simulink library "CryoDetLibCMB"  (R2016b)
settings: Solver=VariableStepAuto  StartTime=0.0  StopTime=10.0  RelTol=1e-3
undefined symbols (not defined in the file): A, B, C, D, Fadc, Fclk, PCIN, xlipgetpartsetting
libraries: xbsIndex_r4 x640, CryoDetLibCMB x81, CryoDetLib x2, simulink x1
(part 7 of 12)

== system CryoDetLibCMB/Loop Filter1 ==
  note: loop filter takes frequency word in, creates frequency word out with setpoint frequency, amplitude
  note: loopFilter
      | multi-line feedback block
      | mplement intial frequency, limits, integrator, gain
  note: F out should be Fi + DF
      | where DF is integral of frequency error dF subject to limits and FBen
  note: Saturate dF at +-FBlimit
  valid : Inport
  feedbackPolarity : Inport  Port=2
  feedbackGain : Inport  Port=3
  feedbackLimitHi : Inport  Port=4
  feedbackLimitLo : Inport  Port=5
  freqError : Inport  Port=6
  freqWord : Inport  Port=7
  ch : Inport  Port=8
  reset : Inport  Port=9
  AddSub1 : xbsIndex_r4/AddSub  mode=Addition  use_carryin=off  use_carryout=off  en=off  latency=3  precision=User Defined  arith_type=Unsigned  n_bits=24  bin_pt=24  quantization=Truncate  overflow=Wrap  use_behavioral_HDL=off  hw_selection=Fabric  pipelined=on  dbl_ovrd=off  block_type=addsub
  BitBasher : xbsIndex_r4/BitBasher  bitexpr=out={fbEn, 3'b0, amp, freq}  display_expr=off  sr_1=out  arith_type1=Unsigned  bin_pt1=0  sr_2=2  arith_type2=Unsigned  bin_pt2=0  sr_3=3  arith_type3=Unsigned  bin_pt3=0  sr_4=4  arith_type4=Unsigned  bin_pt4=0  dbl_ovrd=off  block_type=bitbasher
  Concat1 : xbsIndex_r4/Concat  num_inputs=2  dbl_ovrd=off  block_type=concat
  Constant3 : xbsIndex_r4/Constant  const=0  gui_display_data_type=Fixed-point  arith_type=Signed (2's comp)  n_bits=32  bin_pt=30  preci_type=Single  exp_width=8  frac_width=24  explicit_period=off  period=1  equ=P=C  opselect=C  inp2=PCIN>>17  opr=+  inp1=P  carry=CIN  dbl_ovrd=off  block_type=constant
  Convert : xbsIndex_r4/Convert  gui_display_data_type=Fixed-point  arith_type="Signed  (2's comp)"  n_bits=32  bin_pt=30  float_type=Single  exp_bits=8  fraction_bits=24  quantization=Truncate  overflow=Wrap  en=off  latency=0  pipeline=off  dbl_ovrd=off  block_type=convert
  Convert1 : xbsIndex_r4/Convert  gui_display_data_type=Fixed-point  arith_type="Signed  (2's comp)"  n_bits=16  bin_pt=14  float_type=Single  exp_bits=8  fraction_bits=24  quantization=Truncate  overflow=Wrap  en=off  latency=0  pipeline=off  dbl_ovrd=off  block_type=convert
  Convert2 : xbsIndex_r4/Convert  gui_display_data_type=Fixed-point  arith_type="Signed  (2's comp)"  n_bits=48  bin_pt=37  float_type=Single  exp_bits=8  fraction_bits=24  quantization=Truncate  overflow=Wrap  en=off  latency=0  pipeline=off  dbl_ovrd=off  block_type=convert
  Convert3 : xbsIndex_r4/Convert  gui_display_data_type=Fixed-point  arith_type="Signed  (2's comp)"  n_bits=16  bin_pt=15  float_type=Single  exp_bits=8  fraction_bits=24  quantization=Truncate  overflow=Wrap  en=off  latency=0  pipeline=off  dbl_ovrd=off  block_type=convert
  Convert4 : xbsIndex_r4/Convert  gui_display_data_type=Fixed-point  arith_type="Signed  (2's comp)"  n_bits=16  bin_pt=15  float_type=Single  exp_bits=8  fraction_bits=24  quantization=Truncate  overflow=Wrap  en=off  latency=0  pipeline=off  dbl_ovrd=off  block_type=convert
  Convert5 : xbsIndex_r4/Convert  gui_display_data_type=Fixed-point  arith_type="Signed  (2's comp)"  n_bits=24  bin_pt=23  float_type=Single  exp_bits=8  fraction_bits=24  quantization=Truncate  overflow=Wrap  en=off  latency=0  pipeline=off  dbl_ovrd=off  block_type=convert
  "DSP48 Macro 3.0 " : xbsIndex_r4/DSP48 Macro 3.0   dsptype=Target XtremeDSP Slice: DSP48E2  instruction_list=A*B+C  AvailableInstructions=|  show_filtered=on  pipeline_options=Expert  dspimage=?  tier_1=off  tier_2=off  tier_3=off  tier_4=off  tier_5=off  tier_6=off  dreg_1=off  dreg_2=off  dreg_3=off  areg_1=off  areg_2=off  areg_3=on  areg_4=on  breg_1=off  breg_2=off  breg_3=on  breg_4=on  mreg_5=on  concatreg_3=off  concatreg_4=off  concatreg_5=off  creg_1=off  creg_2=off  creg_3=on  creg_4=on  creg_5=on  preg_6=on  cinreg_1=off  cinreg_2=off  cinreg_3=off  cinreg_4=off  cinreg_5=off  opreg_1=off  opreg_2=off  opreg_3=off  opreg_4=off  opreg_5=off  output_properties=Full_Precision  p_width=33  p_binarywidth=30  has_acout=off  has_bcout=off  has_pcout=off  has_carryout=off  has_carrycascout=off  has_ce=off  has_d_ce=off  has_a_ce=off  has_b_ce=off  has_concat_ce=off  has_c_ce=off  has_m_ce=off  has_p_ce=off  has_sel_ce=off  has_sclr=off  has_d_sclr=off  has_a_sclr=off  has_b_sclr=off  has_concat_sclr=off  has_c_sclr=off  has_m_sclr=off  has_p_sclr=off  has_sel_sclr=off  use_dsp48=on  simulation_type=fast_sim  simulation_model=sysgen:xbip_dsp48_macro_v3_0  gui_behaviour=Sysgen  instruction1='#'  ip_name=DSP48 Macro  ip_version=3.0  dsptool_ready=true  ipcore_usecache=true  ipcore_useipmodelcache=true  wrapper_available=true  port_translation_map={ 'ce' => 'en', 'sclr' => 'rst'}  ipcore_latency_function='has_combinational'  structural_sim=false  ipcore_verbose=false  ipcore_port_config={ 'carryin' => { 'arith' => 'ufix', 'binpt' => 0.00000000000, 'width' => 1.00000000000}, 'carrycascin' => { 'arith' => 'ufix', 'binpt' => 0.00000000000, 'width' => 1.00000000000}, 'carrycascout' => { 'arith' => 'ufix', 'binpt' => 0.00000000000, 'width' => 1.00000000000}, 'carryout' => { 'arith' => 'ufix', 'binpt' => 0.00000000000, 'width' => 1.00000000000}}  ipcore_xco_need_fpga_part=true  block_type=xbip_dsp48_macro_v3_0
      | -(A*B+C)
      | -(A*B+C+CARRYIN)
      | -(A*B+CARRYIN)
      | -(C+A*B+CARRYIN)
      | -(P+A*B+CARRYIN)
      | -C+A*B+C
      | -P+A*B+C
      | -P>>17+A*B+C
      | -PCIN+A*B+C
      | -PCIN>>17+A*B+C
      | A*B+C
      | A*B+C+C
      | A*B+C+C+CARRYIN
      | A*B+C+CARRYIN
      | A*B+C+P
      | A*B+C+P+CARRYIN
      | A*B+C+P>>17
      | A*B+C+P>>17+CARRYIN
      | A*B+C+PCIN
      | A*B+C+PCIN+CARRYIN
      | A*B+C+PCIN>>17
      | A*B+C+PCIN>>17+CARRYIN
      | A*B+C-C
      | A*B+C-P
      | A*B+C-P>>17
      | A*B+C-PCIN
      | A*B+C-PCIN>>17
      | A*B+CARRYIN
      | C+A*B+C
      | C+A*B+C+CARRYIN
      | C+A*B+CARRYIN
      | C+C+A*B+CARRYIN
      | C+P+A*B+CARRYIN
      | C+P>>17+A*B+CARRYIN
      | C+PCIN+A*B+CARRYIN
      | C+PCIN>>17+A*B+CARRYIN
      | C-(A*B+C)
      | C-(A*B+C+CARRYIN)
      | C-(A*B+CARRYIN)
      | C-(C+A*B+CARRYIN)
      | C-(P+A*B+CARRYIN)
      | P+A*B+C
      | P+A*B+C+CARRYIN
      | P+A*B+CARRYIN
      | P+C+A*B+CARRYIN
      | P+P+A*B+CARRYIN
      | P+P>>17+A*B+CARRYIN
      | P+PCIN+A*B+CARRYIN
      | P+PCIN>>17+A*B+CARRYIN
      | P-(A*B+C)
      | P-(A*B+C+CARRYIN)
      | P-(A*B+CARRYIN)
      | P-(C+A*B+CARRYIN)
      | P-(P+A*B+CARRYIN)
      | P>>17+A*B+C
      | P>>17+A*B+C+CARRYIN
      | P>>17+A*B+CARRYIN
      | P>>17+C+A*B+CARRYIN
      | P>>17+P+A*B+CARRYIN
      | P>>17-(A*B+C)
      | P>>17-(A*B+C+CARRYIN)
      | P>>17-(A*B+CARRYIN)
      | P>>17-(C+A*B+CARRYIN)
      | P>>17-(P+A*B+CARRYIN)
      | PCIN+A*B+C
      | PCIN+A*B+C+CARRYIN
      | PCIN+A*B+CARRYIN
      | PCIN+C+A*B+CARRYIN
      | PCIN+P+A*B+CARRYIN
      | PCIN-(A*B+C)
      | PCIN-(A*B+C+CARRYIN)
      | PCIN-(A*B+CARRYIN)
      | PCIN-(C+A*B+CARRYIN)
      | PCIN-(P+A*B+CARRYIN)
      | PCIN>>17+A*B+C
      | PCIN>>17+A*B+C+CARRYIN
      | PCIN>>17+A*B+CARRYIN
      | PCIN>>17+C+A*B+CARRYIN
      | PCIN>>17+P+A*B+CARRYIN
      | PCIN>>17-(A*B+C)
      | PCIN>>17-(A*B+C+CARRYIN)
      | PCIN>>17-(A*B+CARRYIN)
      | PCIN>>17-(C+A*B+CARRYIN)
      | PCIN>>17-(P+A*B+CARRYIN)
      | RNDMACC(A*B+C+P)
      | RNDSIMPLE(A*B+C)
      | RNDSIMPLE(A*B+C+CARRYIN)
      | RNDSIMPLE(A*B+CARRYIN)
      | RNDSIMPLE(C+A*B+CARRYIN)
      | RNDSIMPLE(P+A*B+CARRYIN)
      | RNDSIMPLE(P>>17+A*B+CARRYIN)
      | RNDSIMPLE(PCIN+A*B+CARRYIN)
      | RNDSIMPLE(PCIN>>17+A*B+CARRYIN)
      settings: infoedit=<html>Valid operands: CONCAT, P, C, PCIN, P>>17, PCIN>>17, CARRYIN, CARRYCASCIN, ACIN, A, BCIN,B<br><br>Valid operators: +, -, *, ()<br><br>Valid functions: RNDSIMPLE, RNDSYM<br><br>Instructions are case insensitive and tolerate spaces.</html>
  Delay : xbsIndex_r4/Delay  rst=off  infoeditControl=Selection of Reset will increase slice count due to use of real FFs and instead of SRLs  en=off  latency=121  reg_retiming=off  dbl_ovrd=off  block_type=delay
  Delay1 : xbsIndex_r4/Delay  rst=off  infoeditControl=Selection of Reset will increase slice count due to use of real FFs and instead of SRLs  en=off  latency=4  reg_retiming=off  dbl_ovrd=off  block_type=delay
  Delay2 : xbsIndex_r4/Delay  rst=off  infoeditControl=Selection of Reset will increase slice count due to use of real FFs and instead of SRLs  en=off  latency=3  reg_retiming=off  dbl_ovrd=off  block_type=delay
  Delay3 : xbsIndex_r4/Delay  rst=off  infoeditControl=Selection of Reset will increase slice count due to use of real FFs and instead of SRLs  en=off  latency=3  reg_retiming=off  dbl_ovrd=off  block_type=delay
  Delay4 : xbsIndex_r4/Delay  rst=off  infoeditControl=Selection of Reset will increase slice count due to use of real FFs and instead of SRLs  en=off  latency=3  reg_retiming=off  dbl_ovrd=off  block_type=delay
  Delay7 : xbsIndex_r4/Delay  rst=off  infoeditControl=Selection of Reset will increase slice count due to use of real FFs and instead of SRLs  en=off  latency=10  reg_retiming=off  dbl_ovrd=off  block_type=delay
  Delay8 : xbsIndex_r4/Delay  rst=off  infoeditControl=Selection of Reset will increase slice count due to use of real FFs and instead of SRLs  en=off  latency=10  reg_retiming=off  dbl_ovrd=off  block_type=delay
  Mux : xbsIndex_r4/Mux  inputs=2  en=off  latency=1  precision=User Defined  arith_type="Signed  (2's comp)"  n_bits=16  bin_pt=14  quantization=Truncate  overflow=Wrap  dbl_ovrd=off  block_type=mux
  Mux1 : xbsIndex_r4/Mux  inputs=2  en=off  latency=1  precision=Full  arith_type=Unsigned  n_bits=16  bin_pt=14  quantization=Truncate  overflow=Wrap  dbl_ovrd=off  block_type=mux
  Mux2 : xbsIndex_r4/Mux  inputs=3  en=off  latency=1  precision=Full  arith_type=Unsigned  n_bits=16  bin_pt=14  quantization=Truncate  overflow=Wrap  dbl_ovrd=off  block_type=mux
  Negate : xbsIndex_r4/Negate  precision=User Defined  arith_type="Signed  (2's comp)"  n_bits=16  bin_pt=15  quantization=Truncate  overflow=Wrap  en=off  latency=2  dbl_ovrd=off  block_type=negate
  Register3 : xbsIndex_r4/Register  init=0  rst=off  en=off  dbl_ovrd=off  block_type=register
  Relational3 : xbsIndex_r4/Relational  mode=a>b  op_type=Bool  en=off  latency=1  dbl_ovrd=off  block_type=relational
  Relational4 : xbsIndex_r4/Relational  mode=a<b  op_type=Bool  en=off  latency=1  dbl_ovrd=off  block_type=relational
  freqWordDecoder1 : CryoDetLibCMB/freqWordDecoder
  freqWordDecoder2 : CryoDetLibCMB/freqWordDecoder
  valid_o : Outport
  freqWordOut : Outport  Port=2
  ch_o : Outport  Port=3
  wires:
  Convert5/1 -> "DSP48 Macro 3.0 "/1
  freqError/1 -> Convert5/1
  Mux/1 -> "DSP48 Macro 3.0 "/2
  Convert4/1 -> Mux2/3, Relational4/1
  Convert3/1 -> Relational3/1, Mux2/4
  Convert1/1 -> Mux/2, Negate/1
  "DSP48 Macro 3.0 "/1 -> Convert/1
  Convert2/1 -> "DSP48 Macro 3.0 "/3
  Mux1/1 -> Relational3/2, Relational4/2, Register3/1
  Delay/1 -> Convert2/1
  Mux2/1 -> AddSub1/2, Delay/1
  Register3/1 -> Mux2/2
  feedbackLimitLo/1 -> Convert3/1
  Concat1/1 -> Mux2/1
  Relational4/1 -> Concat1/2
  Relational3/1 -> Concat1/1
  Constant3/1 -> Mux1/2
  Convert/1 -> Mux1/3
  freqWordDecoder1/1 -> Mux1/1
  Negate/1 -> Mux/3
  feedbackLimitHi/1 -> Convert4/1
  feedbackGain/1 -> Convert1/1
  feedbackPolarity/1 -> Mux/1
  freqWord/1 -> Delay1/1
  ch/1 -> Delay7/1
  valid/1 -> Delay8/1
  Delay1/1 -> Delay2/1, freqWordDecoder1/1
  Delay8/1 -> valid_o/1
  Delay7/1 -> ch_o/1
  Delay2/1 -> freqWordDecoder2/1
  freqWordDecoder2/3 -> AddSub1/1
  freqWordDecoder2/2 -> Delay3/1
  freqWordDecoder2/1 -> Delay4/1
  AddSub1/1 -> BitBasher/3  "Fi"
  Delay3/1 -> BitBasher/1
  Delay4/1 -> BitBasher/2
  BitBasher/1 -> freqWordOut/1

== system CryoDetLibCMB/Notch ==
  note: Notch Filter with center angular frequency w0, finite Q, and notch depth
  In : Inport
  w0 : Inport  Port=2
  Gain : Gain  Gain=depth
  Gain1 : Gain  Gain=1/Q
  Integrator1 : Integrator
  Integrator4 : Integrator
  Product : Product
  Product1 : Product
  Sum1 : Sum  Inputs=++|
  Sum2 : Sum  Inputs=|+-
  Sum3 : Sum  Inputs=-+|
  out : Outport
  wires:
  Gain1/1 -> Gain/1, Sum1/1
  Sum2/1 -> Integrator1/1
  In/1 -> Sum2/1, Sum3/2
  w0/1 -> Product/1, Product1/1
  Integrator1/1 -> Product/2
  Product/1 -> Integrator4/1, Gain1/1
  Gain/1 -> Sum3/1
  Sum1/1 -> Sum2/2
  Sum3/1 -> out/1
  Product1/1 -> Sum1/2
  Integrator4/1 -> Product1/2

== system CryoDetLibCMB/Subsystem ==
  note: Interleave DDS phases for 16 channels
      | add registers to aid timing
  In1 : Inport
  In2 : Inport  Port=2
  In3 : Inport  Port=3
  In4 : Inport  Port=4
  In5 : Inport  Port=5
  In6 : Inport  Port=6
  In7 : Inport  Port=7
  In8 : Inport  Port=8
  In9 : Inport  Port=9
  In10 : Inport  Port=10
  In11 : Inport  Port=11
  In12 : Inport  Port=12
  In13 : Inport  Port=13
  In14 : Inport  Port=14
  In15 : Inport  Port=15
  In16 : Inport  Port=16
  BitBasher : xbsIndex_r4/BitBasher  bitexpr=|  display_expr=on  sr_1=hi  arith_type1=Unsigned  bin_pt1=0  sr_2=lo  arith_type2=Unsigned  bin_pt2=0  sr_3=3  arith_type3=Unsigned  bin_pt3=0  sr_4=4  arith_type4=Unsigned  bin_pt4=0  dbl_ovrd=off  block_type=bitbasher
      | hi = {in[3:2]}
      | lo = {in[1:0]}
  Bus Creator : BusCreator  Inputs=2
  Counter : xbsIndex_r4/Counter  cnt_type=Free Running  cnt_to=Inf  operation=Up  start_count=0  cnt_by_val=1  arith_type=Unsigned  n_bits=4  bin_pt=0  load_pin=off  rst=off  en=off  explicit_period=on  period=Tclk  use_behavioral_HDL=off  implementation=Fabric  dbl_ovrd=off  block_type=counter
  Mux{0..4} (5 alike) : xbsIndex_r4/Mux  inputs=4  en=off  latency=1  precision=Full  arith_type=Unsigned  n_bits=16  bin_pt=14  quantization=Truncate  overflow=Wrap  dbl_ovrd=off  block_type=mux
  Register{0..3} (4 alike) : xbsIndex_r4/Register  init=0  rst=off  en=off  dbl_ovrd=off  block_type=register
  Ref : Outport
  wires:
  In13/1 -> Mux3/2
  In6/1 -> Mux1/3
  Mux0/1 -> Mux4/2
  BitBasher/2 -> Mux1/1, Mux2/1, Mux3/1, Mux0/1
  In8/1 -> Mux1/5
  In10/1 -> Mux2/3
  In3/1 -> Mux0/4
  In14/1 -> Mux3/3
  BitBasher/1 -> Register0/1
  In9/1 -> Mux2/2
  In11/1 -> Mux2/4
  Mux1/1 -> Mux4/3
  In2/1 -> Mux0/3
  In15/1 -> Mux3/4
  In4/1 -> Mux0/5
  Mux3/1 -> Mux4/5
  In1/1 -> Mux0/2
  In5/1 -> Mux1/2
  In12/1 -> Mux2/5
  Register0/1 -> Register1/1, Mux4/1
  In7/1 -> Mux1/4
  Counter/1 -> BitBasher/1
  Mux2/1 -> Mux4/4
  Mux4/1 -> Register3/1
  In16/1 -> Mux3/5
  Register3/1 -> Bus Creator/2  "DDS Ref"
  Bus Creator/1 -> Ref/1
  Register2/1 -> Bus Creator/1  "channel"
  Register1/1 -> Register2/1

== system CryoDetLibCMB/amplitude_scale ==
  note: Scale in approx 3 dB steps
      | 4 bits in
      | 0 ==> unscaled
      | 15==> OFF
      | else scale by ~ 2^(-ampl/2)
  valid : Inport
  ampl : Inport  Port=2
  in : Inport  Port=3
  ch : Inport  Port=4
  AddSub : xbsIndex_r4/AddSub  mode=Subtraction  use_carryin=off  use_carryout=off  en=off  latency=2  precision=User Defined  arith_type="Signed  (2's comp)"  n_bits=18  bin_pt=17  quantization=Truncate  overflow=Wrap  use_behavioral_HDL=off  hw_selection=Fabric  pipelined=on  dbl_ovrd=off  block_type=addsub
  BitBasher : xbsIndex_r4/BitBasher  bitexpr=|  display_expr=on  sr_1=frac  arith_type1=Unsigned  bin_pt1=0  sr_2=int  arith_type2=Unsigned  bin_pt2=0  sr_3=int  arith_type3=Unsigned  bin_pt3=0  sr_4=4  arith_type4=Unsigned  bin_pt4=0  dbl_ovrd=off  block_type=bitbasher
      | frac = {ampl[0:0]}
      | int = {ampl[3:1]}
  Constant : xbsIndex_r4/Constant  const=0  gui_display_data_type=Fixed-point  arith_type=Unsigned  n_bits=4  bin_pt=0  preci_type=Single  exp_width=8  frac_width=24  explicit_period=off  period=1  equ=P=C  opselect=C  inp2=PCIN>>17  opr=+  inp1=P  carry=CIN  dbl_ovrd=off  block_type=constant
  Constant1 : xbsIndex_r4/Constant  const=0  gui_display_data_type=Fixed-point  arith_type=Signed (2's comp)  n_bits=18  bin_pt=17  preci_type=Single  exp_width=8  frac_width=24  explicit_period=off  period=1  equ=P=C  opselect=C  inp2=PCIN>>17  opr=+  inp1=P  carry=CIN  dbl_ovrd=off  block_type=constant
  Convert : xbsIndex_r4/Convert  gui_display_data_type=Fixed-point  arith_type="Signed  (2's comp)"  n_bits=18  bin_pt=17  float_type=Single  exp_bits=8  fraction_bits=24  quantization=Truncate  overflow=Wrap  en=off  latency=0  pipeline=off  dbl_ovrd=off  block_type=convert
  Delay : xbsIndex_r4/Delay  rst=off  infoeditControl=Selection of Reset will increase slice count due to use of real FFs and instead of SRLs  en=off  latency=4  reg_retiming=on  dbl_ovrd=off  block_type=delay
  Delay1 : xbsIndex_r4/Delay  rst=off  infoeditControl=Selection of Reset will increase slice count due to use of real FFs and instead of SRLs  en=off  latency=4  reg_retiming=on  dbl_ovrd=off  block_type=delay
  Delay2 : xbsIndex_r4/Delay  rst=off  infoeditControl=Selection of Reset will increase slice count due to use of real FFs and instead of SRLs  en=off  latency=3  reg_retiming=off  dbl_ovrd=off  block_type=delay
  Delay3 : xbsIndex_r4/Delay  rst=off  infoeditControl=Selection of Reset will increase slice count due to use of real FFs and instead of SRLs  en=off  latency=2  reg_retiming=off  dbl_ovrd=off  block_type=delay
  Mux : xbsIndex_r4/Mux  inputs=8  en=off  latency=1  precision=Full  arith_type=Unsigned  n_bits=16  bin_pt=14  quantization=Truncate  overflow=Wrap  dbl_ovrd=off  block_type=mux
  Mux1 : xbsIndex_r4/Mux  inputs=2  en=off  latency=0  precision=Full  arith_type=Unsigned  n_bits=16  bin_pt=14  quantization=Truncate  overflow=Wrap  dbl_ovrd=off  block_type=mux
  Mux2 : xbsIndex_r4/Mux  inputs=2  en=off  latency=1  precision=User Defined  arith_type="Signed  (2's comp)"  n_bits=18  bin_pt=17  quantization=Truncate  overflow=Wrap  dbl_ovrd=off  block_type=mux
  Register2 : xbsIndex_r4/Register  init=0  rst=off  en=off  dbl_ovrd=off  block_type=register
  Register7 : xbsIndex_r4/Register  init=0  rst=off  en=off  dbl_ovrd=off  block_type=register
  Relational : xbsIndex_r4/Relational  mode=a=b  op_type=Bool  en=off  latency=1  dbl_ovrd=off  block_type=relational
  Shift : xbsIndex_r4/Shift  shift_dir=Right  shift_bits=1  en=off  latency=0  precision=User Defined  arith_type="Signed  (2's comp)"  n_bits=18  bin_pt=17  quantization=Truncate  overflow=Wrap  dbl_ovrd=off  block_type=shift
  Shift1 : xbsIndex_r4/Shift  shift_dir=Right  shift_bits=2  en=off  latency=0  precision=User Defined  arith_type="Signed  (2's comp)"  n_bits=18  bin_pt=17  quantization=Truncate  overflow=Wrap  dbl_ovrd=off  block_type=shift
  Shift2 : xbsIndex_r4/Shift  shift_dir=Right  shift_bits=3  en=off  latency=0  precision=User Defined  arith_type="Signed  (2's comp)"  n_bits=18  bin_pt=17  quantization=Truncate  overflow=Wrap  dbl_ovrd=off  block_type=shift
  Shift3 : xbsIndex_r4/Shift  shift_dir=Right  shift_bits=4  en=off  latency=0  precision=User Defined  arith_type="Signed  (2's comp)"  n_bits=18  bin_pt=17  quantization=Truncate  overflow=Wrap  dbl_ovrd=off  block_type=shift
  Shift4 : xbsIndex_r4/Shift  shift_dir=Right  shift_bits=5  en=off  latency=0  precision=User Defined  arith_type="Signed  (2's comp)"  n_bits=18  bin_pt=17  quantization=Truncate  overflow=Wrap  dbl_ovrd=off  block_type=shift
  Shift5 : xbsIndex_r4/Shift  shift_dir=Right  shift_bits=6  en=off  latency=0  precision=User Defined  arith_type="Signed  (2's comp)"  n_bits=18  bin_pt=17  quantization=Truncate  overflow=Wrap  dbl_ovrd=off  block_type=shift
  Shift6 : xbsIndex_r4/Shift  shift_dir=Right  shift_bits=7  en=off  latency=0  precision=User Defined  arith_type="Signed  (2's comp)"  n_bits=18  bin_pt=17  quantization=Truncate  overflow=Wrap  dbl_ovrd=off  block_type=shift
  Shift7 : xbsIndex_r4/Shift  shift_dir=Right  shift_bits=2  en=off  latency=0  precision=User Defined  arith_type="Signed  (2's comp)"  n_bits=18  bin_pt=17  quantization=Truncate  overflow=Wrap  dbl_ovrd=off  block_type=shift
  valid_o : Outport
  out : Outport  Port=2
  ch_o : Outport  Port=3
  wires:
  Delay3/1 -> Mux2/1
  Delay2/1 -> Mux1/1
  Relational/1 -> Delay3/1
  Constant1/1 -> Mux2/3
  Mux2/1 -> out/1
  Mux1/1 -> Mux2/2
  Register2/1 -> Register7/1
  in/1 -> Shift6/1, Shift5/1, Shift4/1, Shift3/1, Shift2/1, Shift1/1, Shift/1, Convert/1
  Constant/1 -> Relational/1
  ampl/1 -> Relational/2, BitBasher/1
  Shift7/1 -> AddSub/2
  Mux/1 -> AddSub/1, Shift7/1, Register2/1
  BitBasher/2 -> Mux/1
  BitBasher/1 -> Delay2/1
  ch/1 -> Delay/1
  Delay/1 -> ch_o/1
  valid/1 -> Delay1/1
  Delay1/1 -> valid_o/1
  Shift1/1 -> Mux/7
  Shift6/1 -> Mux/2
  Shift3/1 -> Mux/5
  Shift/1 -> Mux/8
  Shift4/1 -> Mux/4
  Shift2/1 -> Mux/6
  Shift5/1 -> Mux/3
  Convert/1 -> Mux/9
  AddSub/1 -> Mux1/2
  Register7/1 -> Mux1/3

== system CryoDetLibCMB/confgi0_r ==
  in : Inport
  BitBasher : xbsIndex_r4/BitBasher  bitexpr=|  display_expr=off  sr_1=sel  arith_type1=Unsigned  bin_pt1=0  sr_2=start  arith_type2=Unsigned  bin_pt2=0  sr_3=rf_enable  arith_type3=Unsigned  bin_pt3=0  sr_4=fb_enable  arith_type4=Unsigned  bin_pt4=0  dbl_ovrd=off  block_type=bitbasher
      | sel={in[0]}
      | start={in[1]}
      | rf_enable = {in[2]}
  rf_enable : Outport
  sig_gen_sel : Outport  Port=2
  sig_gen_start : Outport  Port=3
  wires:
  BitBasher/3 -> rf_enable/1
  in/1 -> BitBasher/1
  BitBasher/2 -> sig_gen_start/1
  BitBasher/1 -> sig_gen_sel/1

== system CryoDetLibCMB/config1_r ==
  in : Inport
  BitBasher1 : xbsIndex_r4/BitBasher  bitexpr=|  display_expr=off  sr_1=out_iq_swap  arith_type1=Unsigned  bin_pt1=0  sr_2=in_iq_swap  arith_type2=Unsigned  bin_pt2=0  sr_3=3  arith_type3=Unsigned  bin_pt3=0  sr_4=4  arith_type4=Unsigned  bin_pt4=0  dbl_ovrd=off  block_type=bitbasher
      | out_iq_swap = {in[0]}
      | in_iq_swap = {in[1]}
  out_iq_swap : Outport
  in_iq_swap : Outport  Port=2
  wires:
  in/1 -> BitBasher1/1
  BitBasher1/1 -> out_iq_swap/1  "out_iq_swap"
  BitBasher1/2 -> in_iq_swap/1  "in_iq_swap"

== system CryoDetLibCMB/config2_r ==
  In1 : Inport
  BitBasher : xbsIndex_r4/BitBasher  bitexpr=|  display_expr=off  sr_1=ref_delay  arith_type1=Unsigned  bin_pt1=0  sr_2=tone_scale_sel  arith_type2=Unsigned  bin_pt2=0  sr_3=fb_enable  arith_type3=Unsigned  bin_pt3=0  sr_4=fb_polarity  arith_type4=Unsigned  bin_pt4=0  dbl_ovrd=off  block_type=bitbasher
      | ref_delay = {in[2:0]}
      | tone_scale_sel = {in[4:3]}
      | fb_enable = {in[5]}
      | fb_polarity = {in[6]}
  BitBasher1 : xbsIndex_r4/BitBasher  bitexpr=|  display_expr=off  sr_1=iq_swap_sel  arith_type1=Unsigned  bin_pt1=0  sr_2=iq_band_sel  arith_type2=Unsigned  bin_pt2=0  sr_3=iq_ch_sel  arith_type3=Unsigned  bin_pt3=0  sr_4=fb_polarity  arith_type4=Unsigned  bin_pt4=0  dbl_ovrd=off  block_type=bitbasher
      | iq_swap_sel = {in[7]}
      | iq_band_sel = {in[16:15]}
      | iq_ch_sel = {in[14:8]}
  ref_delay : Outport
  tone_scale_sel : Outport  Port=2
  fb_enable : Outport  Port=3
  fb_polarity : Outport  Port=4
  iq_swap_sel : Outport  Port=5
  iq_band_sel : Outport  Port=6
  iq_ch_sel : Outport  Port=7
  wires:
  In1/1 -> BitBasher1/1, BitBasher/1
  BitBasher/1 -> ref_delay/1
  BitBasher/2 -> tone_scale_sel/1
  BitBasher/3 -> fb_enable/1
  BitBasher/4 -> fb_polarity/1
  BitBasher1/1 -> iq_swap_sel/1
  BitBasher1/2 -> iq_band_sel/1
  BitBasher1/3 -> iq_ch_sel/1

== system CryoDetLibCMB/config3_r ==
  In1 : Inport
  BitBasher1 : xbsIndex_r4/BitBasher  bitexpr=|  display_expr=off  sr_1=fb_gain  arith_type1=Unsigned  bin_pt1=10  sr_2=fb_limit  arith_type2=Unsigned  bin_pt2=16  sr_3=ref_delay  arith_type3=Unsigned  bin_pt3=0  sr_4=4  arith_type4=Unsigned  bin_pt4=0  dbl_ovrd=off  block_type=bitbasher
      | fb_gain = {in[15:0]}
      | fb_limit = {in[31:16]}
  fb_gain : Outport
  fb_limit : Outport  Port=2
  wires:
  BitBasher1/1 -> fb_gain/1
  In1/1 -> BitBasher1/1
  BitBasher1/2 -> fb_limit/1

== system CryoDetLibCMB/dF ==
  note: Check to see if it should be real or imag component!!!
  note: latency 1
  note: Assume I&Q inputs are format 18_16,
      | check and scale, trim, etc to match Fix_18_16
  note: I/Q swap negates sense of rotation
  note: need eta registers reconfigured, etaRAM?
  note: add eta phase then rotate demodulated signal, take one component
  note: definition of eta' changed so that now delta(F) = real part of eta'*Sig*conj(Ref)
      | SS 27 Spe 2017
  note: diagnostics
  note: dF1
  note: Frequency error dF = Re(eta'*Ref'*Sig)
      | where eta' is like a phase and amplitude calibration including the phase determined by the 2 sidebands and amplitude determined by the reference central line and bandwidth
      |
      | get channel ID
      | fetch eta'
      | calc dF
  demod : Inport
  ref phase : Inport  Port=2
  AddSub : xbsIndex_r4/AddSub  mode=Addition  use_carryin=off  use_carryout=off  en=off  latency=3  precision=User Defined  arith_type=Unsigned  n_bits=18  bin_pt=15  quantization=Truncate  overflow=Wrap  use_behavioral_HDL=off  hw_selection=Fabric  pipelined=off  dbl_ovrd=off  block_type=addsub
  Bus Selector : BusSelector  OutputSignals=SignalQ&I.sigQ,SignalQ&I.sigI,channel
  Bus Selector1 : BusSelector  OutputSignals=ref phase,chan
  Bus Selector4 : BusSelector  OutputSignals=etaMag,etaPhase
  Bus Creator : BusCreator  Inputs=2
  "CORDIC 6.0 " : xbsIndex_r4/CORDIC 6.0   functional_selection=Rotate  architectural_configuration=Parallel  pipelining_mode=Optimal  data_format=SignedFraction  phase_format=Scaled_Radians  input_width=17  output_width=18  round_mode=Truncate  iterations=0  precision=0  compensation_scaling=No_Scale_Compensation  coarse_rotation=on  aclken=off  aresetn=off  out_tready=off  cartesian_has_tuser=on  cartesian_has_tlast=off  cartesian_tuser_width=16  phase_has_tuser=on  phase_has_tlast=off  phase_tuser_width=4  out_tlast_behv=Null  flow_control=NonBlocking  optimize_goal=Resources  trim_axipin_name=on  simulation_type=hybrid_sim  simulation_model=sysgen:cordic_v6_0  data_path_portlist={'s_axis_cartesian_tdata_imag', 's_axis_cartesian_tdata_real', 's_axis_phase_tdata_phase', 'm_axis_dout_tdata_imag', 'm_axis_dout_tdata_real', 'm_axis_dout_tdata_phase','m_axis_dout_tdata'}  ip_name=CORDIC  ip_version=6.0  dsptool_ready=true  ipcore_usecache=true  ipcore_useipmodelcache=true  wrapper_available=true  port_translation_map={ 'aclken' => 'en', 'aresetn' => 'rst' }  block_type=cordic_v6_0
      settings: infoedit=CORDIC 6.0
  Constant2 : xbsIndex_r4/Constant  const=1  gui_display_data_type=Boolean  arith_type=Boolean  n_bits=16  bin_pt=14  preci_type=Single  exp_width=8  frac_width=24  explicit_period=off  period=1  equ=P=C  opselect=C  inp2=PCIN>>17  opr=+  inp1=P  carry=CIN  dbl_ovrd=off  block_type=constant
  Constant3 : xbsIndex_r4/Constant  const=0  gui_display_data_type=Fixed-point  arith_type=Unsigned  n_bits=4  bin_pt=0  preci_type=Single  exp_width=8  frac_width=24  explicit_period=off  period=1  equ=P=C  opselect=C  inp2=PCIN>>17  opr=+  inp1=P  carry=CIN  dbl_ovrd=off  block_type=constant
  Convert : xbsIndex_r4/Convert  gui_display_data_type=Fixed-point  arith_type="Signed  (2's comp)"  n_bits=18  bin_pt=16  float_type=Single  exp_bits=8  fraction_bits=24  quantization=Truncate  overflow=Saturate  en=off  latency=1  pipeline=off  dbl_ovrd=off  block_type=convert
  Convert1 : xbsIndex_r4/Convert  gui_display_data_type=Fixed-point  arith_type="Signed  (2's comp)"  n_bits=18  bin_pt=16  float_type=Single  exp_bits=8  fraction_bits=24  quantization=Truncate  overflow=Saturate  en=off  latency=1  pipeline=off  dbl_ovrd=off  block_type=convert
  Delay4 : xbsIndex_r4/Delay  rst=off  infoeditControl=Selection of Reset will increase slice count due to use of real FFs and instead of SRLs  en=off  latency=3  reg_retiming=on  dbl_ovrd=off  block_type=delay
  Delay9 : xbsIndex_r4/Delay  rst=off  infoeditControl=Selection of Reset will increase slice count due to use of real FFs and instead of SRLs  en=off  latency=3  reg_retiming=on  dbl_ovrd=off  block_type=delay
  Gateway Out{1,3,5..8} (6 alike) : xbsIndex_r4/Gateway Out  inherit_from_input=off  hdl_port=off  rows=1  columns=1  UseAsDAC=off  DACChannel='1'  interface=None  automatic_assignment=on  address_offset=hex2dec('00')  intf_name=''  intf_description=''  timing_constraint=None  locs_specified=off  LOCs={}  io_standard={}  block_type=gatewayout
  Im dF : Display
  Mult : xbsIndex_r4/Mult  precision=Full  arith_type="Signed  (2's comp)"  n_bits=16  bin_pt=14  quantization=Truncate  overflow=Wrap  en=off  latency=3  use_behavioral_HDL=off  opt=Speed  use_embedded=on  optimum_pipeline=off  pipeline=on  dbl_ovrd=off  use_rpm=on  placement_style=Triangular  block_type=mult
  Mult1 : xbsIndex_r4/Mult  precision=Full  arith_type="Signed  (2's comp)"  n_bits=16  bin_pt=14  quantization=Truncate  overflow=Wrap  en=off  latency=3  use_behavioral_HDL=off  opt=Speed  use_embedded=on  optimum_pipeline=off  pipeline=on  dbl_ovrd=off  use_rpm=on  placement_style=Triangular  block_type=mult
  Mux : Mux  Inputs=2
  Re dF : Display
  Register2 : xbsIndex_r4/Register  init=0  rst=off  en=on  dbl_ovrd=off  block_type=register
  Register3 : xbsIndex_r4/Register  init=0  rst=off  en=on  dbl_ovrd=off  block_type=register
  Relational2 : xbsIndex_r4/Relational  mode=a=b  op_type=Bool  en=off  latency=0  dbl_ovrd=off  block_type=relational
  Terminator2 : Terminator
  "dF1scope " : Scope  NumInputPorts=3
  dFscope : Scope  NumInputPorts=2
  eta Mux : Subsystem
  ref phase RAM : Subsystem
  ref phase diff : Subsystem
  dF : Outport
  wires:
  demod/1 -> Bus Selector/1
  Bus Selector/3 -> eta Mux/1(channel), ref phase RAM/2(read channel)  "<channel>"
  eta Mux/1(eta out) -> Bus Selector4/1
  Constant3/1 -> Relational2/2
  Relational2/1 -> Register3/2, Register2/2
  Register2/1 -> Gateway Out5/1
  Gateway Out5/1 -> dFscope/1, Re dF/1
  Gateway Out6/1 -> dFscope/2, Im dF/1
  Register3/1 -> Gateway Out6/1
  "CORDIC 6.0 "/1 -> Terminator2/1
  Gateway Out3/1 -> "dF1scope "/1
  ref phase/1 -> ref phase diff/1(ref phase)
  ref phase diff/1(phase diff) -> ref phase RAM/1(ref Phase)
  AddSub/1 -> "CORDIC 6.0 "/6
  Bus Selector/1 -> Convert/1  "<sigQ>"
  Bus Selector4/2 -> AddSub/1  "<etaPhase>"
  ref phase RAM/1(ref phase) -> Bus Selector1/1
  Bus Selector1/1 -> AddSub/2  "<ref phase>"
  Bus Selector1/2 -> "CORDIC 6.0 "/7  "<chan>"
  Delay4/1 -> "CORDIC 6.0 "/3
  Delay9/1 -> "CORDIC 6.0 "/2
  Bus Selector4/1 -> "CORDIC 6.0 "/4  "<etaMag>"
  Constant2/1 -> "CORDIC 6.0 "/5, "CORDIC 6.0 "/1
  "CORDIC 6.0 "/4 -> Mult1/2, Gateway Out3/1, Mult/2  "magEta"
  "CORDIC 6.0 "/3 -> Mult/1  "I"
  "CORDIC 6.0 "/2 -> Mult1/1  "Q"
  Convert/1 -> Delay4/1
  Convert1/1 -> Delay9/1
  Bus Selector/2 -> Convert1/1  "<sigI>"
  Mux/1 -> "dF1scope "/2
  Gateway Out1/1 -> Mux/1
  Gateway Out7/1 -> Mux/2
  Gateway Out8/1 -> "dF1scope "/3
  Mult1/1 -> Register3/1, Gateway Out1/1
  Mult/1 -> Register2/1, Gateway Out7/1, Bus Creator/2  "freqError"
  "CORDIC 6.0 "/5 -> Relational2/1, Gateway Out8/1, Bus Creator/1  "channel"
  Bus Creator/1 -> dF/1
